simulink model "pidinputtheeta"  (R2014a)
settings: Solver=ode45  StartTime=0.0  StopTime=500  RelTol=1e-3
settings Model: Creator=aman  LastModifiedBy=aman

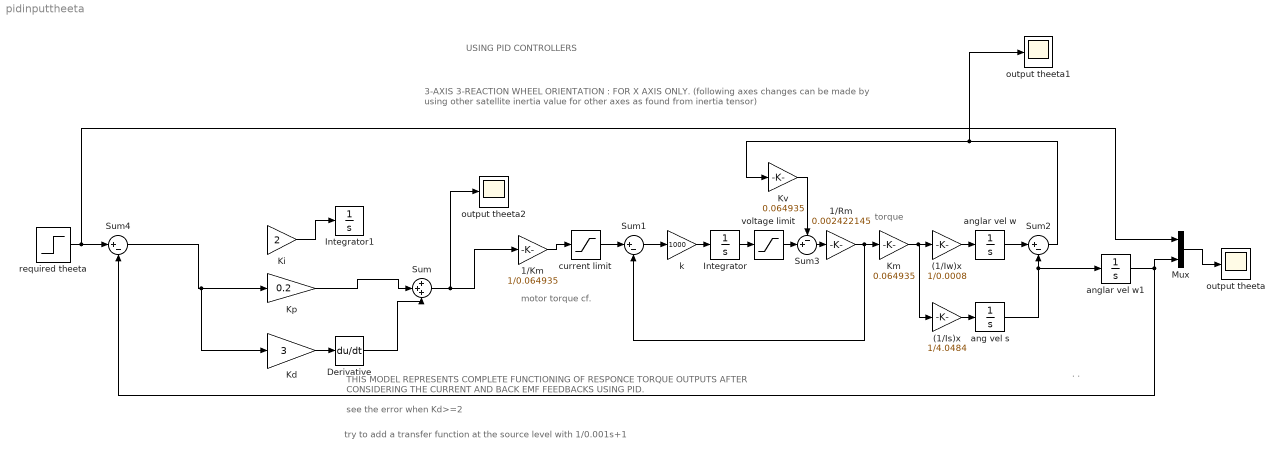
== system pidinputtheeta ==
  note: .
      |
      | .
  note: try to add a transfer function at the source level with 1/0.001s+1
  note: see the error when Kd>=2
  note: USING PID CONTROLLERS
  note: 3-AXIS 3-REACTION WHEEL ORIENTATION : FOR X AXIS ONLY.
      | (following axes changes can be made by using other satellite inertia value for other axes as found from inertia tensor)
  note: torque
  note: THIS MODEL REPRESENTS COMPLETE FUNCTIONING OF RESPONCE TORQUE OUTPUTS AFTER CONSIDERING THE CURRENT AND BACK EMF FEEDBACKS USING PID.
  note: motor
      | torque
      | cf.
  (1/Is)x : Gain  Gain=1/4.0484
  (1/Iw)x : Gain  Gain=1/0.0008
  1/Km : Gain  Gain=1/0.064935
  1/Rm : Gain  Gain=0.002422145
  Derivative : Derivative
  Integrator : Integrator
  Integrator1 : Integrator
  Kd : Gain  Gain=3
  Ki : Gain  Gain=2
  Km : Gain  Gain=0.064935
  Kp : Gain  Gain=0.2
  Kv : Gain  Gain=0.064935
  Mux : Mux  Inputs=2
  Sum : Sum  Inputs=+++
  Sum1 : Sum  Inputs=|+-
  Sum2 : Sum  Inputs=|+-
  Sum3 : Sum  Inputs=-+|
  Sum4 : Sum  Inputs=|+-
  ang vel s : Integrator
  anglar vel w : Integrator
  anglar vel w1 : Integrator
  current limit : Saturate  UpperLimit=0.0816  LowerLimit=-0.016
  k : Gain  Gain=1000
  output theeta : Scope
  output theeta1 : Scope
  output theeta2 : Scope
      settings: SaveName=ScopeData2
  required theeta : Step  After=0.1  SampleTime=0
  voltage limit : Saturate  UpperLimit=34  LowerLimit=-34
  wires:
  1/Km/1 -> current limit/1
  k/1 -> Integrator/1
  Integrator/1 -> voltage limit/1
  1/Rm/1 -> Sum1/2, Km/1
  current limit/1 -> Sum1/1
  Sum1/1 -> k/1
  anglar vel w/1 -> Sum2/1
  (1/Iw)x/1 -> anglar vel w/1
  (1/Is)x/1 -> ang vel s/1
  Km/1 -> (1/Is)x/1, (1/Iw)x/1
  Sum2/1 -> output theeta1/1, Kv/1
  Sum3/1 -> 1/Rm/1
  voltage limit/1 -> Sum3/2
  Kv/1 -> Sum3/1
  Mux/1 -> output theeta/1
  anglar vel w1/1 -> Sum4/2, Mux/2
  Sum/1 -> output theeta2/1, 1/Km/1
  Ki/1 -> Integrator1/1
  Kd/1 -> Derivative/1
  Kp/1 -> Sum/2
  Derivative/1 -> Sum/3
  Sum4/1 -> Kd/1, Kp/1
  required theeta/1 -> Mux/1, Sum4/1
  ang vel s/1 -> anglar vel w1/1, Sum2/2
